simulink subsystem "propellerModel"  (R2023b)
settings: Solver=VariableStepAuto  StartTime=0.0  StopTime=10.0  RelTol=1e-3
undefined symbols (not defined in the file): C_Q0, C_Q1, C_Q2, C_T0, C_T1, C_T2, D_prop, i0, KQ, KV, R_motor, rho, V_max
settings Model: Creator=Victor  LastModifiedBy=Victor

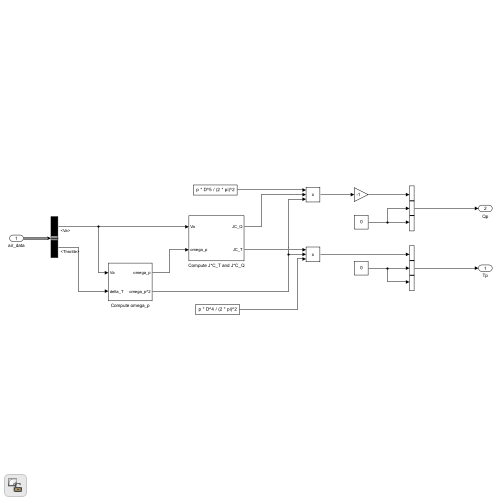
[thumbnail: Simulink's stored preview of the top-level diagram]
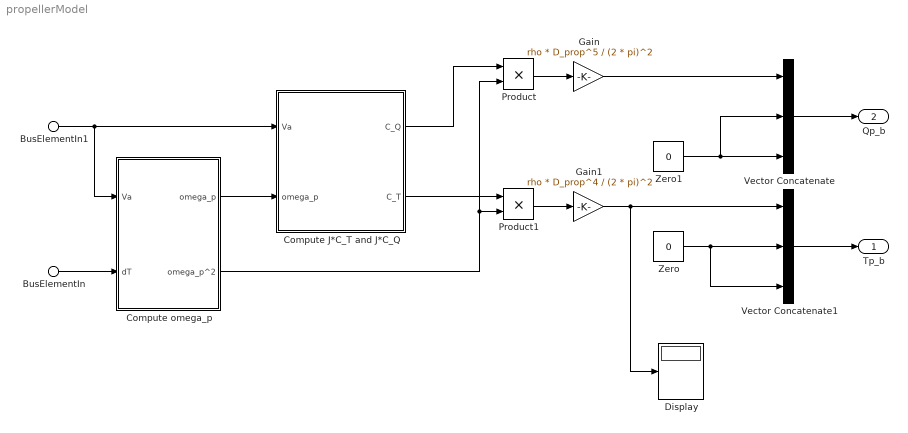
== system propellerModel ==
  BusElementIn : Inport  PortName=uavBus  Element=controlBus.dT
  BusElementIn1 : Inport  PortName=uavBus  Element=targetBus.Va
  Compute J*C_T and J*C_Q : Subsystem
  Compute omega_p : Subsystem
  Display : Display
  Gain : Gain  Gain=rho * D_prop^5 / (2 * pi)^2
  Gain1 : Gain  Gain=rho * D_prop^4 / (2 * pi)^2
  Product : Product
  Product1 : Product
  Vector Concatenate : Concatenate  NumInputs=3
  Vector Concatenate1 : Concatenate  NumInputs=3
  Zero : Constant  Value=0  OutDataTypeStr=Inherit: Inherit via back propagation
  Zero1 : Constant  Value=0  OutDataTypeStr=Inherit: Inherit via back propagation
  Tp_b : Outport
  Qp_b : Outport  Port=2
  wires:
  Compute J*C_T and J*C_Q/1(C_Q) -> Product/1
  Compute J*C_T and J*C_Q/2(C_T) -> Product1/1
  Compute omega_p/1(omega_p) -> Compute J*C_T and J*C_Q/2(omega_p)
  Compute omega_p/2(omega_p^2) -> Product1/2, Product/2
  Gain1/1 -> Display/1, Vector Concatenate1/1
  Gain/1 -> Vector Concatenate/1
  Zero1/1 -> Vector Concatenate/3, Vector Concatenate/2
  Zero/1 -> Vector Concatenate1/2, Vector Concatenate1/3
  BusElementIn1/1 -> Compute omega_p/1(Va), Compute J*C_T and J*C_Q/1(Va)
  BusElementIn/1 -> Compute omega_p/2(dT)
  Product/1 -> Gain/1
  Product1/1 -> Gain1/1
  Vector Concatenate/1 -> Qp_b/1
  Vector Concatenate1/1 -> Tp_b/1

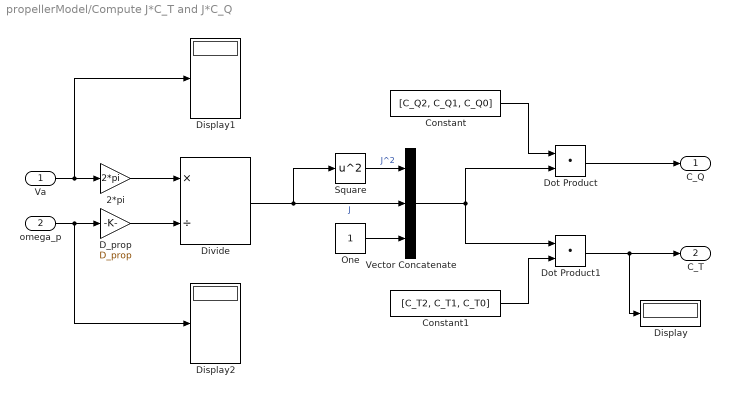
== system propellerModel/Compute J*C_T and J*C_Q ==
  Va : Inport
  omega_p : Inport  Port=2
  2*pi : Gain  Gain=2*pi
  Constant : Constant  Value=[C_Q2, C_Q1, C_Q0]
  Constant1 : Constant  Value=[C_T2, C_T1, C_T0]
  D_prop : Gain  Gain=D_prop
  Display : Display
  Display1 : Display
  Display2 : Display
  Divide : Product  Inputs=*/
  Dot Product : DotProduct  OutDataTypeStr=Inherit: Inherit via internal rule
  Dot Product1 : DotProduct  OutDataTypeStr=Inherit: Inherit via internal rule
  One : Constant  OutDataTypeStr=Inherit: Inherit via back propagation
  Square : Math  Operator=square
  Vector Concatenate : Concatenate  NumInputs=3
  C_Q : Outport
  C_T : Outport  Port=2
  wires:
  2*pi/1 -> Divide/1
  D_prop/1 -> Divide/2
  Va/1 -> 2*pi/1, Display1/1
  omega_p/1 -> D_prop/1, Display2/1
  Divide/1 -> Square/1, Vector Concatenate/2  "J"
  Square/1 -> Vector Concatenate/1  "J^2"
  One/1 -> Vector Concatenate/3
  Constant/1 -> Dot Product/1
  Vector Concatenate/1 -> Dot Product/2, Dot Product1/1
  Constant1/1 -> Dot Product1/2
  Dot Product1/1 -> C_T/1, Display/1
  Dot Product/1 -> C_Q/1

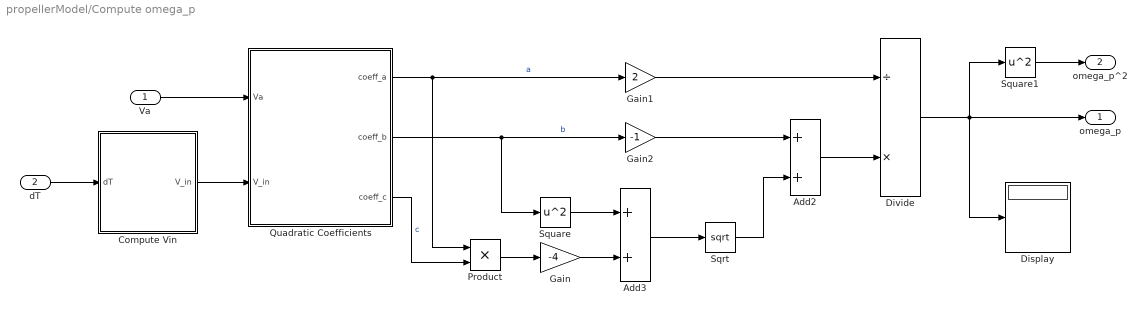
== system propellerModel/Compute omega_p ==
  Va : Inport
  dT : Inport  Port=2
  Add2 : Sum
  Add3 : Sum
  Compute Vin : Subsystem
  Display : Display
  Divide : Product  Inputs=/*
  Gain : Gain  Gain=-4
  Gain1 : Gain  Gain=2
  Gain2 : Gain  Gain=-1
  Product : Product
  Quadratic Coefficients : Subsystem
  Sqrt : Sqrt
  Square : Math  Operator=square
  Square1 : Math  Operator=square
  omega_p : Outport
  omega_p^2 : Outport  Port=2
  wires:
  dT/1 -> Compute Vin/1(dT)
  Product/1 -> Gain/1
  Divide/1 -> Square1/1, Display/1, omega_p/1
  Va/1 -> Quadratic Coefficients/1(Va)
  Compute Vin/1(V_in) -> Quadratic Coefficients/2(V_in)
  Square1/1 -> omega_p^2/1
  Quadratic Coefficients/1(coeff_a) -> Product/1, Gain1/1  "a"
  Gain1/1 -> Divide/1
  Quadratic Coefficients/2(coeff_b) -> Square/1, Gain2/1  "b"
  Gain2/1 -> Add2/1
  Sqrt/1 -> Add2/2
  Add3/1 -> Sqrt/1
  Square/1 -> Add3/1
  Gain/1 -> Add3/2
  Quadratic Coefficients/3(coeff_c) -> Product/2  "c"
  Add2/1 -> Divide/2

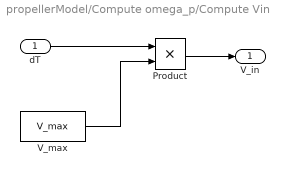
== system propellerModel/Compute omega_p/Compute Vin ==
  dT : Inport
  Product : Product
  V_max : Constant  Value=V_max
  V_in : Outport
  wires:
  V_max/1 -> Product/2
  Product/1 -> V_in/1
  dT/1 -> Product/1

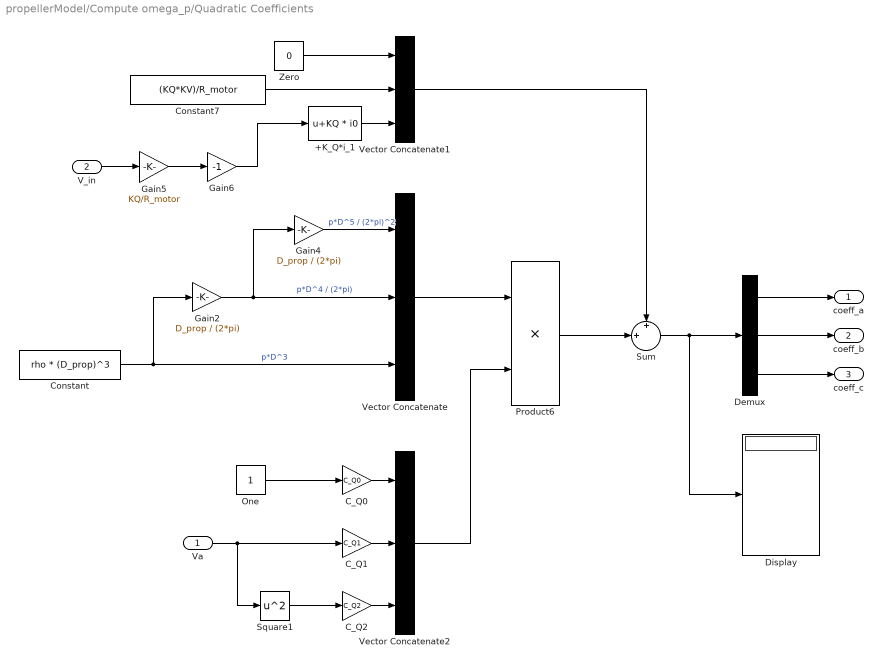
== system propellerModel/Compute omega_p/Quadratic Coefficients ==
  Va : Inport
  V_in : Inport  Port=2
  +K_Q*i_1 : Bias  Bias=KQ * i0  SaturateOnIntegerOverflow=off
  C_Q0 : Gain  Gain=C_Q0
  C_Q1 : Gain  Gain=C_Q1
  C_Q2 : Gain  Gain=C_Q2
  Constant : Constant  Value=rho * (D_prop)^3
  Constant7 : Constant  Value=(KQ*KV)/R_motor
  Demux : Demux  Outputs=3
  Display : Display
  Gain2 : Gain  Gain=D_prop / (2*pi)
  Gain4 : Gain  Gain=D_prop / (2*pi)
  Gain5 : Gain  Gain=KQ/R_motor
  Gain6 : Gain  Gain=-1
  One : Constant  OutDataTypeStr=Inherit: Inherit via back propagation
  Product6 : Product
  Square1 : Math  Operator=square
  Sum : Sum  Inputs=+|+||
  Vector Concatenate : Concatenate  NumInputs=3
  Vector Concatenate1 : Concatenate  NumInputs=3
  Vector Concatenate2 : Concatenate  NumInputs=3
  Zero : Constant  Value=0  OutDataTypeStr=Inherit: Inherit via back propagation
  coeff_a : Outport
  coeff_b : Outport  Port=2
  coeff_c : Outport  Port=3
  wires:
  C_Q1/1 -> Vector Concatenate2/2
  C_Q2/1 -> Vector Concatenate2/3
  C_Q0/1 -> Vector Concatenate2/1
  Product6/1 -> Sum/2
  Demux/3 -> coeff_c/1
  Demux/2 -> coeff_b/1
  Demux/1 -> coeff_a/1
  Sum/1 -> Demux/1, Display/1
  Vector Concatenate1/1 -> Sum/1
  Gain6/1 -> +K_Q*i_1/1
  Gain5/1 -> Gain6/1
  V_in/1 -> Gain5/1
  +K_Q*i_1/1 -> Vector Concatenate1/3
  Constant7/1 -> Vector Concatenate1/2
  Zero/1 -> Vector Concatenate1/1
  Vector Concatenate2/1 -> Product6/2
  Square1/1 -> C_Q2/1
  Va/1 -> C_Q1/1, Square1/1
  One/1 -> C_Q0/1
  Vector Concatenate/1 -> Product6/1
  Gain4/1 -> Vector Concatenate/1  "p*D^5 / (2*pi)^2"
  Gain2/1 -> Gain4/1, Vector Concatenate/2  "p*D^4 / (2*pi)"
  Constant/1 -> Gain2/1, Vector Concatenate/3  "p*D^3"
